simulink model "simLyapRedesign"  (R2015b)
settings: Solver=VariableStepAuto  StartTime=0.0  StopTime=20  RelTol=1e-3
InitFcn:
  | run lyapRedesign.m
values from neighbouring files (symbols this model uses):
  c_hat = mean(c_p)    [lyapRedesign.m]    (also in smc.m)
  e = (x2_bound)/norm(1-1/theta)    [smc.m]
  g = 9.81    [constants.m]    (also in lyapRedesign.m = -9.81; smc.m = -9.81)
  k1 = 100    [lyapRedesign.m]
  k2 = 20 - b_hat    [lyapRedesign.m]
  l = 0.305    [constants.m]    (also in lyapRedesign.m; smc.m)
  m = 0.1    [constants.m]    (also in lyapRedesign.m = mean(m_p); smc.m = min(m_p))
  rho1 = [abs( (1/c_hat - 1/max(c_p))*a ) abs( (a1-min(b_p))/min(c_p) + (b_hat - a1)/c_hat )]    [smc.m]
  rho2 = (Km*A*(5/2000)/(min(m_p)*l))/min(c_p)    [smc.m]
undefined symbols (not defined in the file or in its folder): a_hat, k
settings Model: Creator=jn  LastModifiedBy=jn

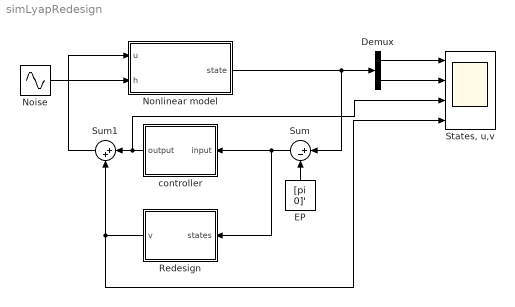
== system simLyapRedesign ==
  Demux : Demux  Outputs=2
  EP : Constant  Value="[pi  0]'"
  Noise : Sin  Frequency=10  SampleTime=0
  Nonlinear model : Subsystem
  Redesign : Subsystem
  "States, u,v" : Scope  NumInputPorts=4
  Sum : Sum  Inputs=|+-
  Sum1 : Sum  Inputs=|++
  controller : Subsystem
  wires:
  Nonlinear model/1(state) -> Demux/1, Sum/1
  Noise/1 -> Nonlinear model/2(h)
  Demux/1 -> "States, u,v"/1
  Demux/2 -> "States, u,v"/2
  Sum/1 -> Redesign/1(states), controller/1(input)
  EP/1 -> Sum/2
  controller/1(output) -> "States, u,v"/3, Sum1/1
  Redesign/1(v) -> "States, u,v"/4, Sum1/2
  Sum1/1 -> Nonlinear model/1(u)

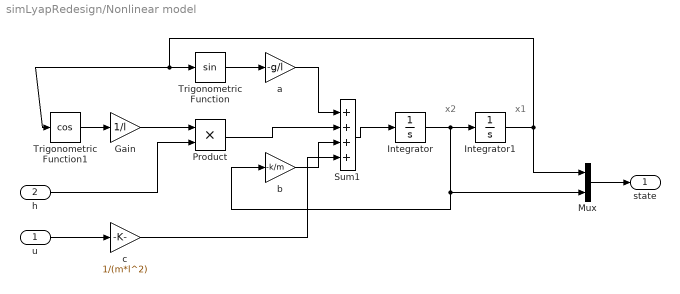
== system simLyapRedesign/Nonlinear model ==
  note: x1
  note: x2
  u : Inport
  h : Inport  Port=2
  Gain : Gain  Gain=1/l
  Integrator : Integrator  ContinuousStateAttributes='speed'
  Integrator1 : Integrator  ContinuousStateAttributes='angle'
  Mux : Mux  Inputs=2
  Product : Product
  Sum1 : Sum  Inputs=++++
  Trigonometric Function : Trigonometry
  Trigonometric Function1 : Trigonometry  Operator=cos
  a : Gain  Gain=-g/l
  b : Gain  Gain=-k/m
  c : Gain  Gain=1/(m*l^2)
  state : Outport
  wires:
  u/1 -> c/1
  Trigonometric Function/1 -> a/1
  a/1 -> Sum1/1
  Sum1/1 -> Integrator/1
  Integrator/1 -> Mux/2, b/1, Integrator1/1
  Integrator1/1 -> Trigonometric Function1/1, Trigonometric Function/1, Mux/1
  Mux/1 -> state/1
  Trigonometric Function1/1 -> Gain/1
  Gain/1 -> Product/1
  h/1 -> Product/2
  Product/1 -> Sum1/2
  b/1 -> Sum1/3
  c/1 -> Sum1/4

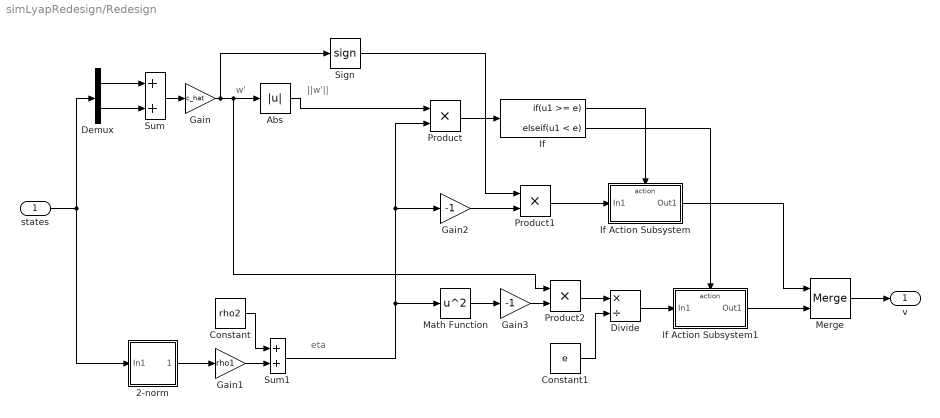
== system simLyapRedesign/Redesign ==
  note: w'
  note: eta
  note: ||w'||
  states : Inport
  2-norm : Subsystem
  Abs : Abs  ZeroCross=off
  Constant : Constant  Value=rho2
  Constant1 : Constant  Value=e
  Demux : Demux  Outputs=2
  Divide : Product  Inputs=*/
  Gain : Gain  Gain=c_hat
  Gain1 : Gain  Gain=rho1
  Gain2 : Gain  Gain=-1
  Gain3 : Gain  Gain=-1
  If : If  IfExpression=u1 >= e  ElseIfExpressions=u1 < e  ShowElse=off  ZeroCross=off
  If Action Subsystem : Subsystem  TreatAsAtomicUnit=on
  If Action Subsystem1 : Subsystem  TreatAsAtomicUnit=on
  Math Function : Math  Operator=square  SaturateOnIntegerOverflow=on
  Merge : Merge
  Product : Product
  Product1 : Product
  Product2 : Product
  Sign : Signum  ZeroCross=off
  Sum : Sum
  Sum1 : Sum
  v : Outport
  wires:
  states/1 -> 2-norm/1(In1), Demux/1
  Demux/2 -> Sum/2
  Demux/1 -> Sum/1
  Sum/1 -> Gain/1
  Gain/1 -> Sign/1, Product2/1, Abs/1
  2-norm/1(Out1) -> Gain1/1
  Gain1/1 -> Sum1/2
  Constant/1 -> Sum1/1
  Sum1/1 -> Gain2/1, Product/2, Math Function/1
  Abs/1 -> Product/1
  Product/1 -> If/1
  If/1 -> If Action Subsystem/Action
  Gain2/1 -> Product1/2
  Sign/1 -> Product1/1
  Product1/1 -> If Action Subsystem/1(In1)
  Merge/1 -> v/1
  If Action Subsystem/1(Out1) -> Merge/1
  Math Function/1 -> Gain3/1
  Gain3/1 -> Product2/2
  Constant1/1 -> Divide/2
  Product2/1 -> Divide/1
  Divide/1 -> If Action Subsystem1/1(In1)
  If Action Subsystem1/1(Out1) -> Merge/2
  If/2 -> If Action Subsystem1/Action

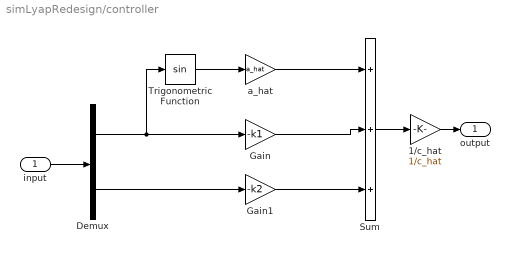
== system simLyapRedesign/controller ==
  input : Inport
  1/c_hat : Gain  Gain=1/c_hat
  Demux : Demux  Outputs=2
  Gain : Gain  Gain=-k1
  Gain1 : Gain  Gain=-k2
  Sum : Sum  Inputs=+++
  Trigonometric Function : Trigonometry
  a_hat : Gain  Gain=a_hat
  output : Outport
  wires:
  input/1 -> Demux/1
  Demux/1 -> Trigonometric Function/1, Gain/1
  Demux/2 -> Gain1/1
  Trigonometric Function/1 -> a_hat/1
  a_hat/1 -> Sum/1
  Gain/1 -> Sum/2
  Gain1/1 -> Sum/3
  1/c_hat/1 -> output/1
  Sum/1 -> 1/c_hat/1

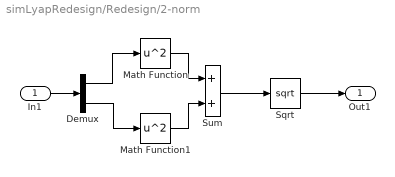
== system simLyapRedesign/Redesign/2-norm ==
  In1 : Inport
  Demux : Demux  Outputs=2
  Math Function : Math  Operator=square  SaturateOnIntegerOverflow=on
  Math Function1 : Math  Operator=square  SaturateOnIntegerOverflow=on
  Sqrt : Sqrt  SaturateOnIntegerOverflow=on
  Sum : Sum
  Out1 : Outport
  wires:
  In1/1 -> Demux/1
  Demux/1 -> Math Function/1
  Demux/2 -> Math Function1/1
  Math Function1/1 -> Sum/2
  Math Function/1 -> Sum/1
  Sum/1 -> Sqrt/1
  Sqrt/1 -> Out1/1

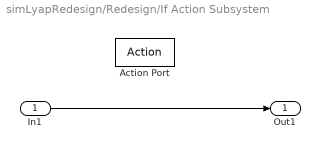
== system simLyapRedesign/Redesign/If Action Subsystem ==
  In1 : Inport
  Action Port : ActionPort  ActionType=then
  Out1 : Outport
  wires:
  In1/1 -> Out1/1

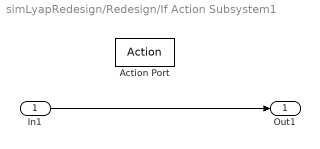
== system simLyapRedesign/Redesign/If Action Subsystem1 ==
  In1 : Inport
  Action Port : ActionPort  ActionType=elseif
  Out1 : Outport
  wires:
  In1/1 -> Out1/1
